simulink model "iscrt"  (R2025a)
settings: Solver=FixedStepDiscrete  StartTime=0.0  StopTime=6  FixedStep=Ts  RelTol=1e-3
model workspace (MATLAB code in the model file):
  | N = 31;
  | n = 0:N-1;
  | sigma = (N-1)/6;
  | g = exp(-0.5*((n-(N-1)/2)/sigma).^2);
  | h = g / sum(g);
undefined symbols (not defined in the file): DiscIntNeverNeededParam, Ts
libraries: simulink x2
settings Model: Creator=wattanakhonvipanna  LastModifiedBy=wattanakhonvipanna

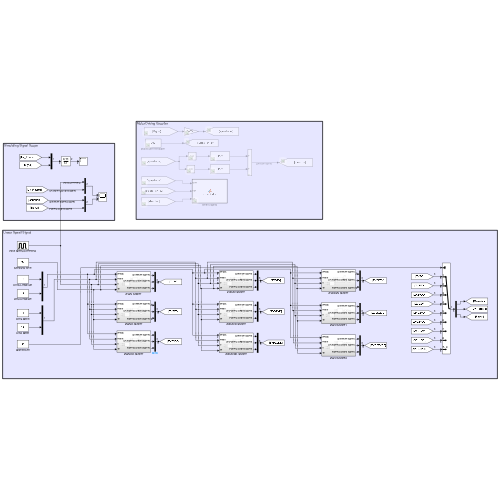
[thumbnail: Simulink's stored preview of the top-level diagram]
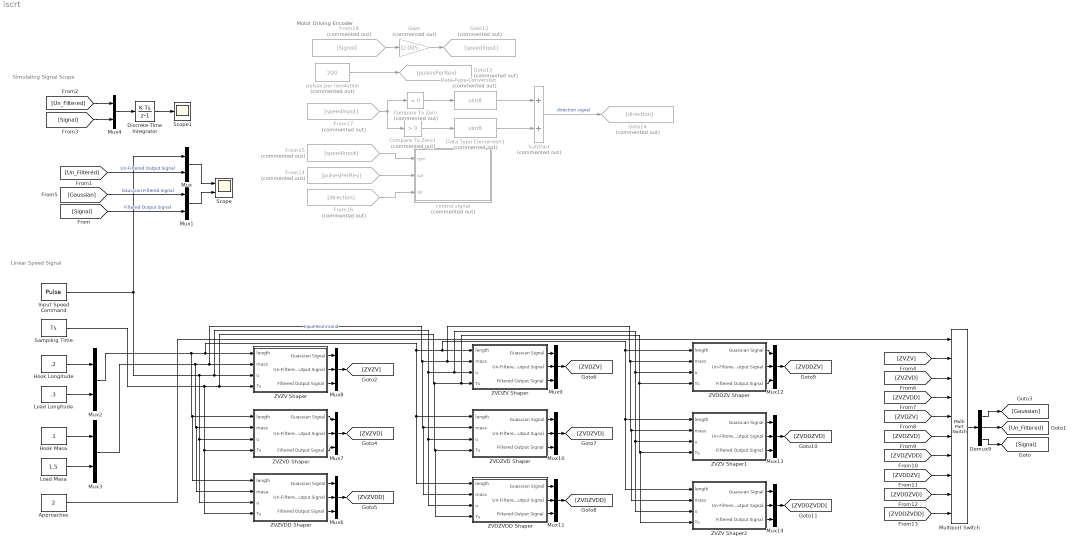
== system iscrt ==
  note: Motor Driving Encoder
  note: Linear Speed Signal
  note: Simulating Signal Scope
  Approaches : Constant  Value=2
  Compare To Zero : simulink/Logic and Bit Operations/Compare To Zero  Commented=on  relop=<  OutDataTypeStr=boolean
  Compare To Zero1 : simulink/Logic and Bit Operations/Compare To Zero  Commented=on  relop=>  OutDataTypeStr=boolean
  Data Type Conversion : DataTypeConversion  Commented=on  OutDataTypeStr=uint8  SaturateOnIntegerOverflow=off  RndMeth=Floor
  Data Type Conversion1 : DataTypeConversion  Commented=on  OutDataTypeStr=uint8  SaturateOnIntegerOverflow=off  RndMeth=Floor
  Demux9 : Demux  Outputs=3
  Discrete-Time Integrator : DiscreteIntegrator  SampleTime=-1  ICPrevOutput=DiscIntNeverNeededParam  ICPrevScaledInput=DiscIntNeverNeededParam
  From14 : From  Commented=on  GotoTag=pulsesPerRev
  From15 : From  Commented=on  GotoTag=speedInput
  From16 : From  Commented=on  GotoTag=direction
  From17 : From  Commented=on  GotoTag=speedInput
  From18 : From  Commented=on  GotoTag=Signal
  Gain : Gain  Commented=on  Gain=1/.005
  Goto12 : Goto  Commented=on  GotoTag=speedInput
  Goto13 : Goto  Commented=on  GotoTag=pulsesPerRev
  Goto14 : Goto  Commented=on  GotoTag=direction
  Hook Longitude : Constant  Value=.2
  Hook Masa : Constant  Value=.1
  Input Speed Command : DiscretePulseGenerator  PulseType=Time based  Amplitude=0.2  Period=10  PulseWidth=50
  Load Longitude : Constant  Value=.3
  Load Masa : Constant  Value=1.5
  Multiport Switch : MultiPortSwitch  Inputs=9  SaturateOnIntegerOverflow=off  InputSameDT=off
  Mux{,1..4} (5 alike) : Mux  Inputs=2
  Mux{6..14} (9 alike) : Mux  Inputs=3
  Sampling Time : Constant  Value=Ts
  Scope : Scope  NumInputPorts=2
      settings: ActiveDisplayYMinimum=-0.024999999999999994  ActiveDisplayYMaximum=0.225  YLabel=speed (m/s)
  Scope1 : Scope
      settings: ActiveDisplayYMinimum=-0.31249999999999656  ActiveDisplayYMaximum=2.8124999999999694  YLabel=position (m)  DataLoggingVariableName=ScopeData2
  Subtract : Sum  Commented=on
  ZVDDZV Shaper : Subsystem
  ZVDZV Shaper : Subsystem
  ZVDZVD Shaper : Subsystem
  ZVDZVDD Shaper : Subsystem
  ZVZV Shaper : Subsystem
  ZVZV Shaper1 : Subsystem
  ZVZV Shaper2 : Subsystem
  ZVZVD Shaper : Subsystem
  ZVZVDD Shaper : Subsystem
  control signal : MATLAB Function  Commented=on  TreatAsAtomicUnit=on
  pulses per revolution : Constant  Commented=on  Value=200
  wires:
  [Un_Filtered] -> Mux/2  "Un-Filtered Output Signal"
  Mux/1 -> Scope/1
  Input Speed Command/1 -> ZVZVDD Shaper/3(u), ZVZVD Shaper/3(u), ZVDZVDD Shaper/3(u), ZVDZVD Shaper/3(u), ZVZV Shaper2/3(u), ZVZV Shaper1/3(u), ZVDDZV Shaper/3(u), ZVDZV Shaper/3(u), ZVZV Shaper/3(u), Mux/1  "Input Command"
  [Gaussian] -> Mux1/1  "Gaussian Filtered Signal"
  [Signal] -> Mux1/2  "Filtered Output Signal"
  Hook Longitude/1 -> Mux2/1
  Load Longitude/1 -> Mux2/2
  Load Masa/1 -> Mux3/2
  Hook Masa/1 -> Mux3/1
  Mux4/1 -> Discrete-Time Integrator/1
  [Un_Filtered] -> Mux4/1
  [Signal] -> Mux4/2
  Discrete-Time Integrator/1 -> Scope1/1
  Mux3/1 -> ZVZVDD Shaper/2(masa), ZVZVD Shaper/2(mass), ZVDZVDD Shaper/2(mass), ZVDZVD Shaper/2(mass), ZVZV Shaper2/2(mass), ZVZV Shaper1/2(mass), ZVDDZV Shaper/2(mass), ZVDZV Shaper/2(mass), ZVZV Shaper/2(mass)
  Sampling Time/1 -> ZVZVDD Shaper/4(Ts), ZVZVD Shaper/4(Ts), ZVDZVDD Shaper/4(Ts), ZVDZVD Shaper/4(Ts), ZVZV Shaper2/4(Ts), ZVZV Shaper1/4(Ts), ZVDDZV Shaper/4(Ts), ZVDZV Shaper/4(Ts), ZVZV Shaper/4(Ts)
  Mux2/1 -> ZVZVDD Shaper/1(length), ZVZVD Shaper/1(length), ZVDZVDD Shaper/1(length), ZVDZVD Shaper/1(length), ZVZV Shaper2/1(length), ZVZV Shaper1/1(length), ZVDDZV Shaper/1(length), ZVDZV Shaper/1(length), ZVZV Shaper/1(length)
  ZVZVDD Shaper/2(Un-Filtered Output Signal) -> Mux6/2
  ZVZVDD Shaper/3(Filtered Output Signal) -> Mux6/3
  ZVZVDD Shaper/1(Guassian Signal) -> Mux6/1
  ZVZVD Shaper/3(Filtered Output Signal) -> Mux7/3
  ZVZVD Shaper/2(Un-Filtered Output Signal) -> Mux7/2
  ZVZVD Shaper/1(Guassian Signal) -> Mux7/1
  ZVZV Shaper/3(Filtered Output Signal) -> Mux8/3
  ZVZV Shaper/2(Un-Filtered Output Signal) -> Mux8/2
  ZVZV Shaper/1(Guassian Signal) -> Mux8/1
  ZVDZV Shaper/3(Filtered Output Signal) -> Mux9/3
  ZVDZV Shaper/2(Un-Filtered Output Signal) -> Mux9/2
  ZVDZV Shaper/1(Guassian Signal) -> Mux9/1
  ZVDZVD Shaper/1(Guassian Signal) -> Mux10/1
  ZVDZVD Shaper/2(Un-Filtered Output Signal) -> Mux10/2
  ZVDZVD Shaper/3(Filtered Output Signal) -> Mux10/3
  ZVDZVDD Shaper/1(Guassian Signal) -> Mux11/1
  ZVDZVDD Shaper/2(Un-Filtered Output Signal) -> Mux11/2
  ZVDZVDD Shaper/3(Filtered Output Signal) -> Mux11/3
  ZVDDZV Shaper/1(Guassian Signal) -> Mux12/1
  ZVDDZV Shaper/2(Un-Filtered Output Signal) -> Mux12/2
  ZVDDZV Shaper/3(Filtered Output Signal) -> Mux12/3
  ZVZV Shaper1/1(Guassian Signal) -> Mux13/1
  ZVZV Shaper1/2(Un-Filtered Output Signal) -> Mux13/2
  ZVZV Shaper1/3(Filtered Output Signal) -> Mux13/3
  ZVZV Shaper2/1(Guassian Signal) -> Mux14/1
  ZVZV Shaper2/2(Un-Filtered Output Signal) -> Mux14/2
  ZVZV Shaper2/3(Filtered Output Signal) -> Mux14/3
  Multiport Switch/1 -> Demux9/1
  Demux9/1 -> [Gaussian]
  Demux9/2 -> [Un_Filtered]
  Demux9/3 -> [Signal]
  Mux8/1 -> [ZVZV]
  Mux7/1 -> [ZVZVD]
  Mux6/1 -> [ZVZVDD]
  Mux9/1 -> [ZVDZV]
  Mux10/1 -> [ZVDZVD]
  Mux11/1 -> [ZVDZVDD]
  Mux12/1 -> [ZVDDZV]
  Mux13/1 -> [ZVDDZVD]
  Mux14/1 -> [ZVDDZVDD]
  [ZVZV] -> Multiport Switch/2
  [ZVZVD] -> Multiport Switch/3
  [ZVZVDD] -> Multiport Switch/4
  [ZVDZV] -> Multiport Switch/5
  [ZVDZVD] -> Multiport Switch/6
  [ZVDZVDD] -> Multiport Switch/7
  [ZVDDZV] -> Multiport Switch/8
  [ZVDDZVD] -> Multiport Switch/9
  [ZVDDZVDD] -> Multiport Switch/10
  Approaches/1 -> Multiport Switch/1
  Data Type Conversion/1 -> Subtract/1
  pulses per revolution/1 -> Goto13/1
  Compare To Zero/1 -> Data Type Conversion/1
  From16/1 -> control signal/3(dir)
  From15/1 -> control signal/1(rpm)
  From14/1 -> control signal/2(spr)
  Data Type Conversion1/1 -> Subtract/2
  From18/1 -> Gain/1
  Subtract/1 -> Goto14/1  "direction signal"
  Compare To Zero1/1 -> Data Type Conversion1/1
  From17/1 -> Compare To Zero/1, Compare To Zero1/1
  Gain/1 -> Goto12/1
  Mux1/1 -> Scope/2

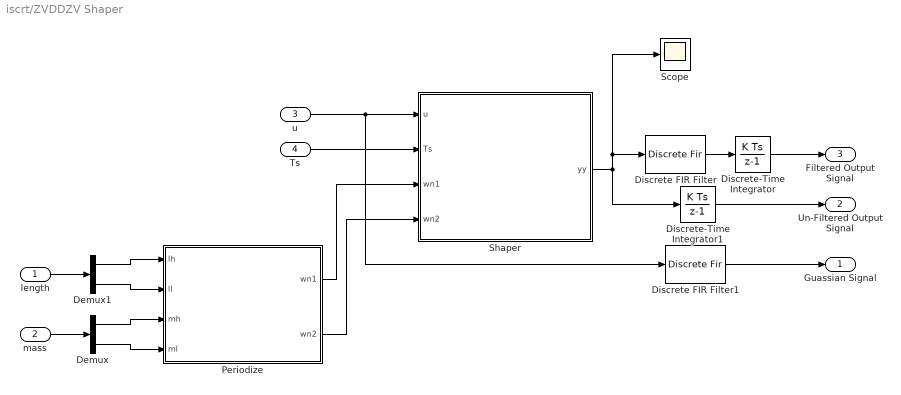
== system iscrt/ZVDDZV Shaper ==
  length : Inport
  mass : Inport  Port=2
  u : Inport  Port=3
  Ts : Inport  Port=4
  Demux : Demux  Outputs=2
  Demux1 : Demux  Outputs=2
  Discrete FIR Filter : DiscreteFir  Coefficients=h
  Discrete FIR Filter1 : DiscreteFir  Coefficients=h
  Discrete-Time Integrator : DiscreteIntegrator  SampleTime=Ts  ICPrevOutput=DiscIntNeverNeededParam  ICPrevScaledInput=DiscIntNeverNeededParam
  Discrete-Time Integrator1 : DiscreteIntegrator  SampleTime=Ts  ICPrevOutput=DiscIntNeverNeededParam  ICPrevScaledInput=DiscIntNeverNeededParam
  Periodize : MATLAB Function  TreatAsAtomicUnit=on
  Scope : Scope
      settings: ActiveDisplayYMinimum=-9993.7500000000018  ActiveDisplayYMaximum=9993.7500000000018  YLabel=Shaper Impulse (ms^-^2)
  Shaper : MATLAB Function  TreatAsAtomicUnit=on
  Guassian Signal : Outport
  Un-Filtered Output Signal : Outport  Port=2
  Filtered Output Signal : Outport  Port=3
  wires:
  Discrete-Time Integrator/1 -> Filtered Output Signal/1
  Shaper/1(yy) -> Discrete-Time Integrator1/1, Scope/1, Discrete FIR Filter/1
  Discrete FIR Filter/1 -> Discrete-Time Integrator/1
  Discrete-Time Integrator1/1 -> Un-Filtered Output Signal/1
  Discrete FIR Filter1/1 -> Guassian Signal/1
  Demux1/1 -> Periodize/1(lh)
  Demux1/2 -> Periodize/2(ll)
  Demux/1 -> Periodize/3(mh)
  Demux/2 -> Periodize/4(ml)
  Periodize/1(wn1) -> Shaper/3(wn1)
  Periodize/2(wn2) -> Shaper/4(wn2)
  mass/1 -> Demux/1
  length/1 -> Demux1/1
  Ts/1 -> Shaper/2(Ts)
  u/1 -> Discrete FIR Filter1/1, Shaper/1(u)

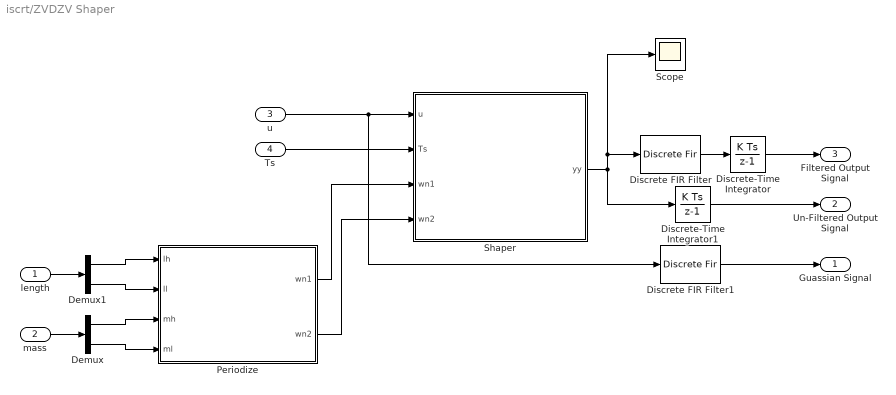
== system iscrt/ZVDZV Shaper ==
  length : Inport
  mass : Inport  Port=2
  u : Inport  Port=3
  Ts : Inport  Port=4
  Demux : Demux  Outputs=2
  Demux1 : Demux  Outputs=2
  Discrete FIR Filter : DiscreteFir  Coefficients=h
  Discrete FIR Filter1 : DiscreteFir  Coefficients=h
  Discrete-Time Integrator : DiscreteIntegrator  SampleTime=Ts  ICPrevOutput=DiscIntNeverNeededParam  ICPrevScaledInput=DiscIntNeverNeededParam
  Discrete-Time Integrator1 : DiscreteIntegrator  SampleTime=Ts  ICPrevOutput=DiscIntNeverNeededParam  ICPrevScaledInput=DiscIntNeverNeededParam
  Periodize : MATLAB Function  TreatAsAtomicUnit=on
  Scope : Scope
      settings: ActiveDisplayYMinimum=-9993.7500000000018  ActiveDisplayYMaximum=9993.7500000000018  YLabel=Shaper Impulse (ms^-^2)
  Shaper : MATLAB Function  TreatAsAtomicUnit=on
  Guassian Signal : Outport
  Un-Filtered Output Signal : Outport  Port=2
  Filtered Output Signal : Outport  Port=3
  wires:
  Discrete-Time Integrator/1 -> Filtered Output Signal/1
  Shaper/1(yy) -> Discrete-Time Integrator1/1, Scope/1, Discrete FIR Filter/1
  Discrete FIR Filter/1 -> Discrete-Time Integrator/1
  Discrete-Time Integrator1/1 -> Un-Filtered Output Signal/1
  Discrete FIR Filter1/1 -> Guassian Signal/1
  Demux1/1 -> Periodize/1(lh)
  Demux1/2 -> Periodize/2(ll)
  Demux/1 -> Periodize/3(mh)
  Demux/2 -> Periodize/4(ml)
  Periodize/1(wn1) -> Shaper/3(wn1)
  Periodize/2(wn2) -> Shaper/4(wn2)
  mass/1 -> Demux/1
  length/1 -> Demux1/1
  Ts/1 -> Shaper/2(Ts)
  u/1 -> Discrete FIR Filter1/1, Shaper/1(u)

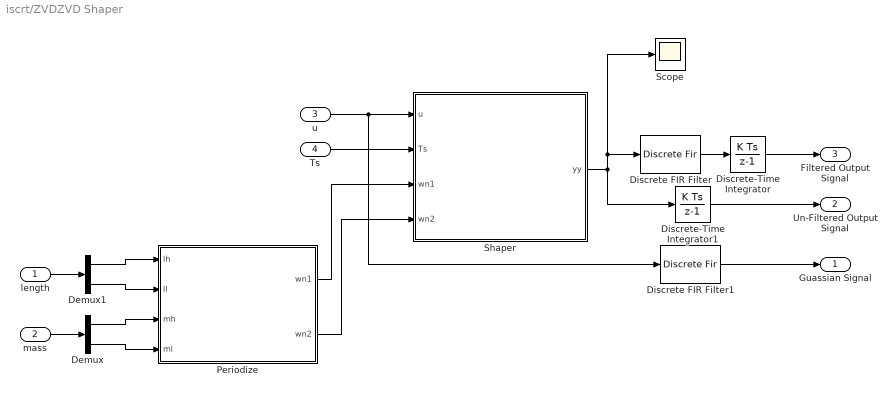
== system iscrt/ZVDZVD Shaper ==
  length : Inport
  mass : Inport  Port=2
  u : Inport  Port=3
  Ts : Inport  Port=4
  Demux : Demux  Outputs=2
  Demux1 : Demux  Outputs=2
  Discrete FIR Filter : DiscreteFir  Coefficients=h
  Discrete FIR Filter1 : DiscreteFir  Coefficients=h
  Discrete-Time Integrator : DiscreteIntegrator  SampleTime=Ts  ICPrevOutput=DiscIntNeverNeededParam  ICPrevScaledInput=DiscIntNeverNeededParam
  Discrete-Time Integrator1 : DiscreteIntegrator  SampleTime=Ts  ICPrevOutput=DiscIntNeverNeededParam  ICPrevScaledInput=DiscIntNeverNeededParam
  Periodize : MATLAB Function  TreatAsAtomicUnit=on
  Scope : Scope
      settings: ActiveDisplayYMinimum=-9993.7500000000018  ActiveDisplayYMaximum=9993.7500000000018  YLabel=Shaper Impulse (ms^-^2)
  Shaper : MATLAB Function  TreatAsAtomicUnit=on
  Guassian Signal : Outport
  Un-Filtered Output Signal : Outport  Port=2
  Filtered Output Signal : Outport  Port=3
  wires:
  Discrete-Time Integrator/1 -> Filtered Output Signal/1
  Shaper/1(yy) -> Discrete-Time Integrator1/1, Scope/1, Discrete FIR Filter/1
  Discrete FIR Filter/1 -> Discrete-Time Integrator/1
  Discrete-Time Integrator1/1 -> Un-Filtered Output Signal/1
  Discrete FIR Filter1/1 -> Guassian Signal/1
  Demux1/1 -> Periodize/1(lh)
  Demux1/2 -> Periodize/2(ll)
  Demux/1 -> Periodize/3(mh)
  Demux/2 -> Periodize/4(ml)
  Periodize/1(wn1) -> Shaper/3(wn1)
  Periodize/2(wn2) -> Shaper/4(wn2)
  length/1 -> Demux1/1
  mass/1 -> Demux/1
  Ts/1 -> Shaper/2(Ts)
  u/1 -> Discrete FIR Filter1/1, Shaper/1(u)

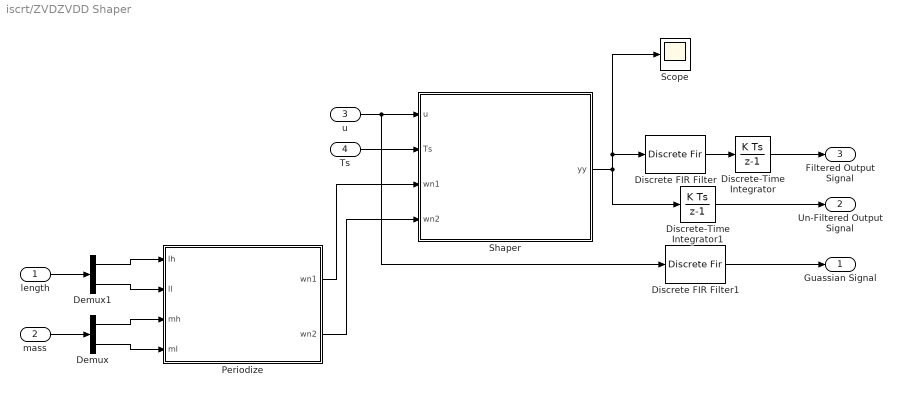
== system iscrt/ZVDZVDD Shaper ==
  length : Inport
  mass : Inport  Port=2
  u : Inport  Port=3
  Ts : Inport  Port=4
  Demux : Demux  Outputs=2
  Demux1 : Demux  Outputs=2
  Discrete FIR Filter : DiscreteFir  Coefficients=h
  Discrete FIR Filter1 : DiscreteFir  Coefficients=h
  Discrete-Time Integrator : DiscreteIntegrator  SampleTime=Ts  ICPrevOutput=DiscIntNeverNeededParam  ICPrevScaledInput=DiscIntNeverNeededParam
  Discrete-Time Integrator1 : DiscreteIntegrator  SampleTime=Ts  ICPrevOutput=DiscIntNeverNeededParam  ICPrevScaledInput=DiscIntNeverNeededParam
  Periodize : MATLAB Function  TreatAsAtomicUnit=on
  Scope : Scope
      settings: ActiveDisplayYMinimum=-9993.7500000000018  ActiveDisplayYMaximum=9993.7500000000018  YLabel=Shaper Impulse (ms^-^2)
  Shaper : MATLAB Function  TreatAsAtomicUnit=on
  Guassian Signal : Outport
  Un-Filtered Output Signal : Outport  Port=2
  Filtered Output Signal : Outport  Port=3
  wires:
  Discrete-Time Integrator/1 -> Filtered Output Signal/1
  Shaper/1(yy) -> Discrete-Time Integrator1/1, Scope/1, Discrete FIR Filter/1
  Discrete FIR Filter/1 -> Discrete-Time Integrator/1
  Discrete-Time Integrator1/1 -> Un-Filtered Output Signal/1
  Discrete FIR Filter1/1 -> Guassian Signal/1
  Demux1/1 -> Periodize/1(lh)
  Demux1/2 -> Periodize/2(ll)
  Demux/1 -> Periodize/3(mh)
  Demux/2 -> Periodize/4(ml)
  Periodize/1(wn1) -> Shaper/3(wn1)
  Periodize/2(wn2) -> Shaper/4(wn2)
  u/1 -> Discrete FIR Filter1/1, Shaper/1(u)
  Ts/1 -> Shaper/2(Ts)
  length/1 -> Demux1/1
  mass/1 -> Demux/1

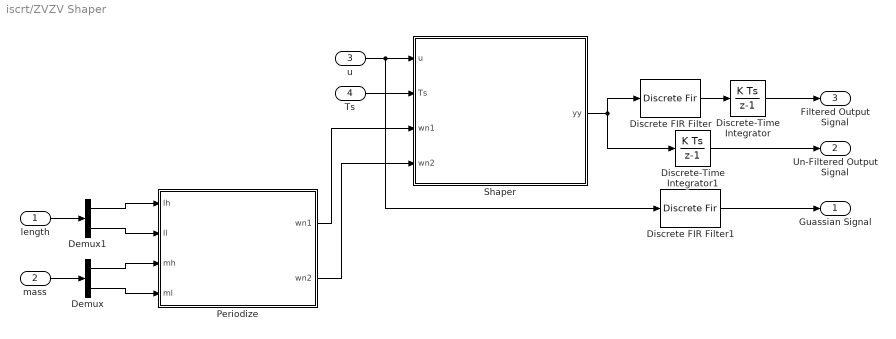
== system iscrt/ZVZV Shaper ==
  length : Inport
  mass : Inport  Port=2
  u : Inport  Port=3
  Ts : Inport  Port=4
  Demux : Demux  Outputs=2
  Demux1 : Demux  Outputs=2
  Discrete FIR Filter : DiscreteFir  Coefficients=h
  Discrete FIR Filter1 : DiscreteFir  Coefficients=h
  Discrete-Time Integrator : DiscreteIntegrator  SampleTime=Ts  ICPrevOutput=DiscIntNeverNeededParam  ICPrevScaledInput=DiscIntNeverNeededParam
  Discrete-Time Integrator1 : DiscreteIntegrator  SampleTime=Ts  ICPrevOutput=DiscIntNeverNeededParam  ICPrevScaledInput=DiscIntNeverNeededParam
  Periodize : MATLAB Function  TreatAsAtomicUnit=on
  Shaper : MATLAB Function  TreatAsAtomicUnit=on
  Guassian Signal : Outport
  Un-Filtered Output Signal : Outport  Port=2
  Filtered Output Signal : Outport  Port=3
  wires:
  Discrete-Time Integrator/1 -> Filtered Output Signal/1
  Shaper/1(yy) -> Discrete-Time Integrator1/1, Discrete FIR Filter/1
  Discrete FIR Filter/1 -> Discrete-Time Integrator/1
  Discrete-Time Integrator1/1 -> Un-Filtered Output Signal/1
  Discrete FIR Filter1/1 -> Guassian Signal/1
  Demux1/1 -> Periodize/1(lh)
  Demux1/2 -> Periodize/2(ll)
  Demux/1 -> Periodize/3(mh)
  Demux/2 -> Periodize/4(ml)
  Periodize/1(wn1) -> Shaper/3(wn1)
  Periodize/2(wn2) -> Shaper/4(wn2)
  length/1 -> Demux1/1
  mass/1 -> Demux/1
  u/1 -> Discrete FIR Filter1/1, Shaper/1(u)
  Ts/1 -> Shaper/2(Ts)

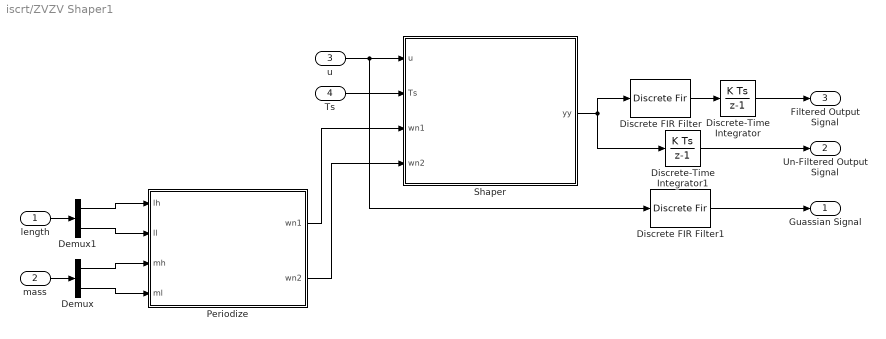
== system iscrt/ZVZV Shaper1 ==
  length : Inport
  mass : Inport  Port=2
  u : Inport  Port=3
  Ts : Inport  Port=4
  Demux : Demux  Outputs=2
  Demux1 : Demux  Outputs=2
  Discrete FIR Filter : DiscreteFir  Coefficients=h
  Discrete FIR Filter1 : DiscreteFir  Coefficients=h
  Discrete-Time Integrator : DiscreteIntegrator  SampleTime=Ts  ICPrevOutput=DiscIntNeverNeededParam  ICPrevScaledInput=DiscIntNeverNeededParam
  Discrete-Time Integrator1 : DiscreteIntegrator  SampleTime=Ts  ICPrevOutput=DiscIntNeverNeededParam  ICPrevScaledInput=DiscIntNeverNeededParam
  Periodize : MATLAB Function  TreatAsAtomicUnit=on
  Shaper : MATLAB Function  TreatAsAtomicUnit=on
  Guassian Signal : Outport
  Un-Filtered Output Signal : Outport  Port=2
  Filtered Output Signal : Outport  Port=3
  wires:
  Discrete-Time Integrator/1 -> Filtered Output Signal/1
  Shaper/1(yy) -> Discrete-Time Integrator1/1, Discrete FIR Filter/1
  Discrete FIR Filter/1 -> Discrete-Time Integrator/1
  Discrete-Time Integrator1/1 -> Un-Filtered Output Signal/1
  Discrete FIR Filter1/1 -> Guassian Signal/1
  Demux1/1 -> Periodize/1(lh)
  Demux1/2 -> Periodize/2(ll)
  Demux/1 -> Periodize/3(mh)
  Demux/2 -> Periodize/4(ml)
  Periodize/1(wn1) -> Shaper/3(wn1)
  Periodize/2(wn2) -> Shaper/4(wn2)
  u/1 -> Discrete FIR Filter1/1, Shaper/1(u)
  Ts/1 -> Shaper/2(Ts)
  mass/1 -> Demux/1
  length/1 -> Demux1/1

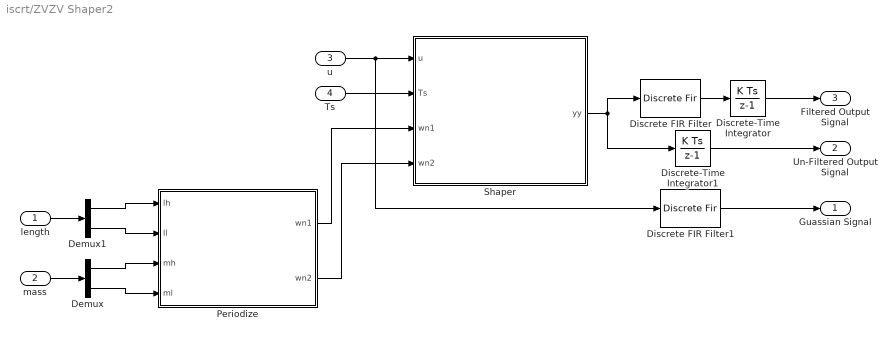
== system iscrt/ZVZV Shaper2 ==
  length : Inport
  mass : Inport  Port=2
  u : Inport  Port=3
  Ts : Inport  Port=4
  Demux : Demux  Outputs=2
  Demux1 : Demux  Outputs=2
  Discrete FIR Filter : DiscreteFir  Coefficients=h
  Discrete FIR Filter1 : DiscreteFir  Coefficients=h
  Discrete-Time Integrator : DiscreteIntegrator  SampleTime=Ts  ICPrevOutput=DiscIntNeverNeededParam  ICPrevScaledInput=DiscIntNeverNeededParam
  Discrete-Time Integrator1 : DiscreteIntegrator  SampleTime=Ts  ICPrevOutput=DiscIntNeverNeededParam  ICPrevScaledInput=DiscIntNeverNeededParam
  Periodize : MATLAB Function  TreatAsAtomicUnit=on
  Shaper : MATLAB Function  TreatAsAtomicUnit=on
  Guassian Signal : Outport
  Un-Filtered Output Signal : Outport  Port=2
  Filtered Output Signal : Outport  Port=3
  wires:
  Discrete-Time Integrator/1 -> Filtered Output Signal/1
  Shaper/1(yy) -> Discrete-Time Integrator1/1, Discrete FIR Filter/1
  Discrete FIR Filter/1 -> Discrete-Time Integrator/1
  Discrete-Time Integrator1/1 -> Un-Filtered Output Signal/1
  Discrete FIR Filter1/1 -> Guassian Signal/1
  Demux1/1 -> Periodize/1(lh)
  Demux1/2 -> Periodize/2(ll)
  Demux/1 -> Periodize/3(mh)
  Demux/2 -> Periodize/4(ml)
  Periodize/1(wn1) -> Shaper/3(wn1)
  Periodize/2(wn2) -> Shaper/4(wn2)
  Ts/1 -> Shaper/2(Ts)
  length/1 -> Demux1/1
  mass/1 -> Demux/1
  u/1 -> Discrete FIR Filter1/1, Shaper/1(u)

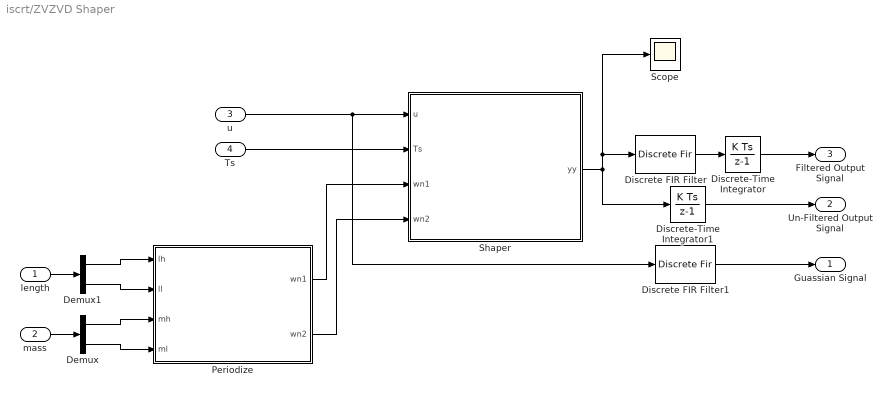
== system iscrt/ZVZVD Shaper ==
  length : Inport
  mass : Inport  Port=2
  u : Inport  Port=3
  Ts : Inport  Port=4
  Demux : Demux  Outputs=2
  Demux1 : Demux  Outputs=2
  Discrete FIR Filter : DiscreteFir  Coefficients=h
  Discrete FIR Filter1 : DiscreteFir  Coefficients=h
  Discrete-Time Integrator : DiscreteIntegrator  SampleTime=Ts  ICPrevOutput=DiscIntNeverNeededParam  ICPrevScaledInput=DiscIntNeverNeededParam
  Discrete-Time Integrator1 : DiscreteIntegrator  SampleTime=Ts  ICPrevOutput=DiscIntNeverNeededParam  ICPrevScaledInput=DiscIntNeverNeededParam
  Periodize : MATLAB Function  TreatAsAtomicUnit=on
  Scope : Scope
      settings: ActiveDisplayYMinimum=-1332.5  ActiveDisplayYMaximum=1332.5  YLabel=Shaper Impulse (ms^-^2)
  Shaper : MATLAB Function  TreatAsAtomicUnit=on
  Guassian Signal : Outport
  Un-Filtered Output Signal : Outport  Port=2
  Filtered Output Signal : Outport  Port=3
  wires:
  Discrete-Time Integrator/1 -> Filtered Output Signal/1
  Shaper/1(yy) -> Discrete-Time Integrator1/1, Scope/1, Discrete FIR Filter/1
  Discrete FIR Filter/1 -> Discrete-Time Integrator/1
  Discrete-Time Integrator1/1 -> Un-Filtered Output Signal/1
  Discrete FIR Filter1/1 -> Guassian Signal/1
  Demux1/1 -> Periodize/1(lh)
  Demux1/2 -> Periodize/2(ll)
  Demux/1 -> Periodize/3(mh)
  Demux/2 -> Periodize/4(ml)
  Periodize/1(wn1) -> Shaper/3(wn1)
  Periodize/2(wn2) -> Shaper/4(wn2)
  mass/1 -> Demux/1
  length/1 -> Demux1/1
  Ts/1 -> Shaper/2(Ts)
  u/1 -> Discrete FIR Filter1/1, Shaper/1(u)

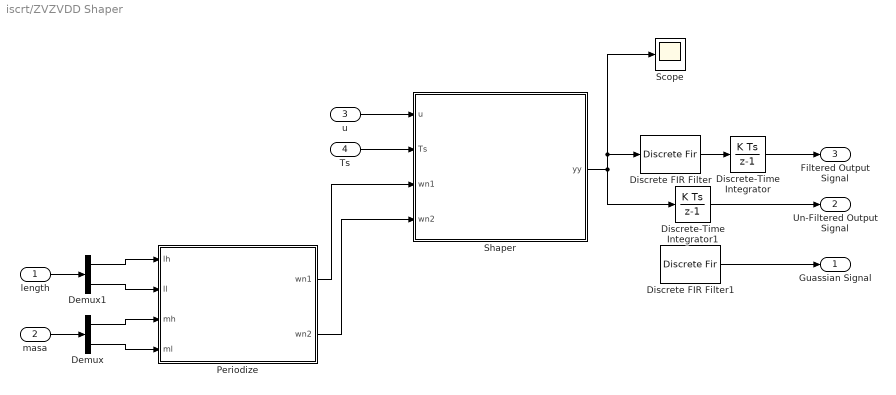
== system iscrt/ZVZVDD Shaper ==
  length : Inport
  masa : Inport  Port=2
  u : Inport  Port=3
  Ts : Inport  Port=4
  Demux : Demux  Outputs=2
  Demux1 : Demux  Outputs=2
  Discrete FIR Filter : DiscreteFir  Coefficients=h
  Discrete FIR Filter1 : DiscreteFir  Coefficients=h
  Discrete-Time Integrator : DiscreteIntegrator  SampleTime=Ts  ICPrevOutput=DiscIntNeverNeededParam  ICPrevScaledInput=DiscIntNeverNeededParam
  Discrete-Time Integrator1 : DiscreteIntegrator  SampleTime=Ts  ICPrevOutput=DiscIntNeverNeededParam  ICPrevScaledInput=DiscIntNeverNeededParam
  Periodize : MATLAB Function  TreatAsAtomicUnit=on
  Scope : Scope
      settings: ActiveDisplayYMinimum=-9993.7500000000018  ActiveDisplayYMaximum=9993.7500000000018  YLabel=Shaper Impulse (ms^-^2)
  Shaper : MATLAB Function  TreatAsAtomicUnit=on
  Guassian Signal : Outport
  Un-Filtered Output Signal : Outport  Port=2
  Filtered Output Signal : Outport  Port=3
  wires:
  Discrete-Time Integrator/1 -> Filtered Output Signal/1
  Shaper/1(yy) -> Discrete-Time Integrator1/1, Scope/1, Discrete FIR Filter/1
  Discrete FIR Filter/1 -> Discrete-Time Integrator/1
  Discrete-Time Integrator1/1 -> Un-Filtered Output Signal/1
  Discrete FIR Filter1/1 -> Guassian Signal/1
  Demux1/1 -> Periodize/1(lh)
  Demux1/2 -> Periodize/2(ll)
  Demux/1 -> Periodize/3(mh)
  Demux/2 -> Periodize/4(ml)
  Periodize/1(wn1) -> Shaper/3(wn1)
  Periodize/2(wn2) -> Shaper/4(wn2)
  masa/1 -> Demux/1
  length/1 -> Demux1/1
  u/1 -> Shaper/1(u)
  Ts/1 -> Shaper/2(Ts)

== matlab function iscrt/ZVDZVD Shaper/Shaper ==
  data: u input; yy output; Ts input; wn1 input; wn2 input
function yy = ZVZVshaper(u, Ts, wn1, wn2)

persistent armed k last_u A_tot d2 d3 d4 d5 d6 d7 d8 d9
if isempty(armed)
    armed  = false;
    k      = double(0);
    last_u = 0.0;
    A_tot  = 0.0;
    d2     = double(0);
    d3     = double(0);
    d4     = double(0);
    d5     = double(0);
    d6     = double(0);
    d7     = double(0);
    d8     = double(0);
    d9     = double(0);
end

yy = 0.0;                
tol = 1e-12;

du = u - last_u;
last_u = u;

if ~armed && (abs(du) > tol)
    A_tot = du;
    k     = double(0);
    T1    = 2*pi / max(wn1, 1e-9);
    T2    = 2*pi / max(wn2, 1e-9);
    d2    = double( round( (0.5*T2) / max(Ts,1e-12) ) ); 
    d3    = double( round( T2 / max(Ts,1e-12) ) );
    d4    = double( round( (0.5*T1) / max(Ts,1e-12) ) );
    d5    = double( round( 0.5*(T1+T2) / max(Ts,1e-12) ) );
    d6    = double( round( (0.5*T1+T2) / max(Ts,1e-12) ) );
    d7    = double( round( T1 / max(Ts,1e-12) ) );
    d8    = double( round( (0.5*T2+T1) / max(Ts,1e-12) ) );
    d9    = double( round( (T2+T1) / max(Ts,1e-12) ) );
    armed = true;
end


if armed
    if k == double(0)
        yy = ((1/16)*A_tot)  / max(Ts,1e-12);
    elseif k == d2
        yy = ((2/16)*A_tot)  / max(Ts,1e-12);
    elseif k == d3
        yy = ((1/16)*A_tot)  / max(Ts,1e-12);
    elseif k == d4
        yy = ((2/16)*A_tot)  / max(Ts,1e-12);
    elseif k == d5
        yy = ((4/16)*A_tot)  / max(Ts,1e-12);
    elseif k == d6
        yy = ((2/16)*A_tot)  / max(Ts,1e-12);
    elseif k == d7
        yy = ((1/16)*A_tot)  / max(Ts,1e-12);
    elseif k == d8
        yy = ((2/16)*A_tot)  / max(Ts,1e-12);
    elseif k == d9
        yy = ((1/16)*A_tot)  / max(Ts,1e-12);
    end

    k = k + double(1);
    if k > d9 + double(1)
        armed = false;
    end
end

== matlab function iscrt/ZVDZVDD Shaper/Periodize ==
  data: lh input; ll input; mh input; wn1 output; wn2 output; ml input
function [wn1, wn2]= ModePeriodize(lh, ll, mh, ml)

g = 9.81;

a = mh * lh * ll;
b = (mh * g * ll) + (ml * g * ll) + (mh * g * lh) + (ml * g * lh);
c = (mh * g * g) + (ml * g * g);

wn1 = sqrt((b - sqrt(b * b - 4 * a * c))/ (2 * a));
wn2 = sqrt((b + sqrt(b * b - 4 * a * c))/ (2 * a));

== matlab function iscrt/ZVDZVDD Shaper/Shaper ==
  data: u input; yy output; Ts input; wn1 input; wn2 input
function yy = ZVZVshaper(u, Ts, wn1, wn2)

persistent armed k last_u A_tot d2 d3 d4 d5 d6 d7 d8 d9 d10 d11 d12
if isempty(armed)
    armed  = false;
    k      = double(0);
    last_u = 0.0;
    A_tot  = 0.0;
    d2     = double(0);
    d3     = double(0);
    d4     = double(0);
    d5     = double(0);
    d6     = double(0);
    d7     = double(0);
    d8     = double(0);
    d9     = double(0);
    d10    = double(0);
    d11    = double(0);
    d12    = double(0);
end

yy = 0.0;                
tol = 1e-12;

du = u - last_u;
last_u = u;

if ~armed && (abs(du) > tol)
    A_tot = du;
    k     = double(0);
    T1    = 2*pi / max(wn1, 1e-9);
    T2    = 2*pi / max(wn2, 1e-9);
    d2    = double( round( (0.5*T2) / max(Ts,1e-12) ) ); 
    d3    = double( round( T2 / max(Ts,1e-12) ) );
    d4    = double( round( (1.5*T2) / max(Ts,1e-12) ) );
    d5    = double( round( (0.5*T1) / max(Ts,1e-12) ) );
    d6    = double( round( 0.5*(T1+T2) / max(Ts,1e-12) ) );
    d7    = double( round( (0.5*T1+T2) / max(Ts,1e-12) ) );
    d8    = double( round( (0.5*T1+1.5*T2) / max(Ts,1e-12) ) );
    d9    = double( round( T1 / max(Ts,1e-12) ) );
    d10   = double( round( (0.5*T2+T1) / max(Ts,1e-12) ) );
    d11   = double( round( (T1+T2) / max(Ts,1e-12) ) );
    d12   = double( round( (T1+1.5*T2) / max(Ts,1e-12) ) );
    armed = true;
end


if armed
    if k == double(0)
        yy = ((1/32)*A_tot)  / max(Ts,1e-12);
    elseif k == d2
        yy = ((3/32)*A_tot)  / max(Ts,1e-12);
    elseif k == d3
        yy = ((3/32)*A_tot)  / max(Ts,1e-12);
    elseif k == d4
        yy = ((1/32)*A_tot)  / max(Ts,1e-12);
    elseif k == d5
        yy = ((2/32)*A_tot)  / max(Ts,1e-12);
    elseif k == d6
        yy = ((6/32)*A_tot)  / max(Ts,1e-12);
    elseif k == d7
        yy = ((6/32)*A_tot)  / max(Ts,1e-12);
    elseif k == d8
        yy = ((2/32)*A_tot)  / max(Ts,1e-12);
    elseif k == d9
        yy = ((1/32)*A_tot)  / max(Ts,1e-12);
    elseif k == d10
        yy = ((3/32)*A_tot)  / max(Ts,1e-12);
    elseif k == d11
        yy = ((3/32)*A_tot)  / max(Ts,1e-12);
    elseif k == d12
        yy = ((1/32)*A_tot)  / max(Ts,1e-12);
    end

    k = k + double(1);
    if k > d12 + double(1)
        armed = false;
    end
end

== matlab function iscrt/ZVZV Shaper/Periodize ==
  data: lh input; ll input; mh input; wn1 output; wn2 output; ml input
function [wn1, wn2]= ModePeriodize(lh, ll, mh, ml)

g = 9.81;

a = mh * lh * ll;
b = (mh * g * ll) + (ml * g * ll) + (mh * g * lh) + (ml * g * lh);
c = (mh * g * g) + (ml * g * g);

wn1 = sqrt((b - sqrt(b * b - 4 * a * c))/ (2 * a));
wn2 = sqrt((b + sqrt(b * b - 4 * a * c))/ (2 * a));

== matlab function iscrt/ZVDDZV Shaper/Periodize ==
  data: lh input; ll input; mh input; wn1 output; wn2 output; ml input
function [wn1, wn2]= ModePeriodize(lh, ll, mh, ml)

g = 9.81;

a = mh * lh * ll;
b = (mh * g * ll) + (ml * g * ll) + (mh * g * lh) + (ml * g * lh);
c = (mh * g * g) + (ml * g * g);

wn1 = sqrt((b - sqrt(b * b - 4 * a * c))/ (2 * a));
wn2 = sqrt((b + sqrt(b * b - 4 * a * c))/ (2 * a));

== matlab function iscrt/ZVDDZV Shaper/Shaper ==
  data: u input; yy output; Ts input; wn1 input; wn2 input
function yy = ZVZVshaper(u, Ts, wn1, wn2)

persistent armed k last_u A_tot d2 d3 d4 d5 d6 d7 d8
if isempty(armed)
    armed  = false;
    k      = double(0);
    last_u = 0.0;
    A_tot  = 0.0;
    d2     = double(0);
    d3     = double(0);
    d4     = double(0);
    d5     = double(0);
    d6     = double(0);
    d7     = double(0);
    d8     = double(0);
end

yy = 0.0;                
tol = 1e-12;

du = u - last_u;
last_u = u;

if ~armed && (abs(du) > tol)
    A_tot = du;
    k     = double(0);
    T1    = 2*pi / max(wn1, 1e-9);
    T2    = 2*pi / max(wn2, 1e-9);
    d2    = double( round( (0.5*T2) / max(Ts,1e-12) ) ); 
    d3    = double( round( (0.5*T1) / max(Ts,1e-12) ) );
    d4    = double( round( 0.5*(T1+T2) / max(Ts,1e-12) ) );
    d5    = double( round( T1 / max(Ts,1e-12) ) );
    d6    = double( round( (0.5*T2+T1) / max(Ts,1e-12) ) );
    d7    = double( round( (1.5*T1) / max(Ts,1e-12) ) );
    d8    = double( round( ((1.5*T1)+(0.5*T2)) / max(Ts,1e-12) ) );
    armed = true;
end


if armed
    if k == double(0)
        yy = ((1/16)*A_tot)  / max(Ts,1e-12);
    elseif k == d2
        yy = ((1/16)*A_tot)  / max(Ts,1e-12);
    elseif k == d3
        yy = ((3/16)*A_tot)  / max(Ts,1e-12);
    elseif k == d4
        yy = ((3/16)*A_tot)  / max(Ts,1e-12);
    elseif k == d5
        yy = ((3/16)*A_tot)  / max(Ts,1e-12);
    elseif k == d6
        yy = ((3/16)*A_tot)  / max(Ts,1e-12);
    elseif k == d7
        yy = ((1/16)*A_tot)  / max(Ts,1e-12);
    elseif k == d8
        yy = ((1/16)*A_tot)  / max(Ts,1e-12);
    end

    k = k + double(1);
    if k > d8 + double(1)
        armed = false;
    end
end

== matlab function iscrt/ZVZV Shaper1/Periodize ==
  data: lh input; ll input; mh input; wn1 output; wn2 output; ml input
function [wn1, wn2]= ModePeriodize(lh, ll, mh, ml)

g = 9.81;

a = mh * lh * ll;
b = (mh * g * ll) + (ml * g * ll) + (mh * g * lh) + (ml * g * lh);
c = (mh * g * g) + (ml * g * g);

wn1 = sqrt((b - sqrt(b * b - 4 * a * c))/ (2 * a));
wn2 = sqrt((b + sqrt(b * b - 4 * a * c))/ (2 * a));

== matlab function iscrt/ZVZV Shaper1/Shaper ==
  data: u input; yy output; Ts input; wn1 input; wn2 input
function yy = ZVZVshaper(u, Ts, wn1, wn2)

persistent armed k last_u A_tot d2 d3 d4 d5 d6 d7 d8 d9 d10 d11 d12
if isempty(armed)
    armed  = false;
    k      = double(0);
    last_u = 0.0;
    A_tot  = 0.0;
    d2     = double(0);
    d3     = double(0);
    d4     = double(0);
    d5     = double(0);
    d6     = double(0);
    d7     = double(0);
    d8     = double(0);
    d9     = double(0);
    d10    = double(0);
    d11    = double(0);
    d12    = double(0);
end

yy = 0.0;                
tol = 1e-12;

du = u - last_u;
last_u = u;

if ~armed && (abs(du) > tol)
    A_tot = du;
    k     = double(0);
    T1    = 2*pi / max(wn1, 1e-9);
    T2    = 2*pi / max(wn2, 1e-9);
    d2    = double( round( (0.5*T2) / max(Ts,1e-12) ) ); 
    d3    = double( round( T2 / max(Ts,1e-12) ) );
    d4    = double( round( (0.5*T1) / max(Ts,1e-12) ) );
    d5    = double( round( 0.5*(T1+T2) / max(Ts,1e-12) ) );
    d6    = double( round( (0.5*T1+T2) / max(Ts,1e-12) ) );
    d7    = double( round( T1 / max(Ts,1e-12) ) );
    d8    = double( round( (T1+0.5*T2) / max(Ts,1e-12) ) );
    d9    = double( round( (T1+T2) / max(Ts,1e-12) ) );
    d10   = double( round( (1.5*T1) / max(Ts,1e-12) ) );
    d11   = double( round( (1.5*T1+0.5*T2) / max(Ts,1e-12) ) );
    d12   = double( round( (1.5*T1+T2) / max(Ts,1e-12) ) );
    armed = true;
end


if armed
    if k == double(0)
        yy = ((1/32)*A_tot)  / max(Ts,1e-12);
    elseif k == d2
        yy = ((2/32)*A_tot)  / max(Ts,1e-12);
    elseif k == d3
        yy = ((1/32)*A_tot)  / max(Ts,1e-12);
    elseif k == d4
        yy = ((3/32)*A_tot)  / max(Ts,1e-12);
    elseif k == d5
        yy = ((6/32)*A_tot)  / max(Ts,1e-12);
    elseif k == d6
        yy = ((3/32)*A_tot)  / max(Ts,1e-12);
    elseif k == d7
        yy = ((3/32)*A_tot)  / max(Ts,1e-12);
    elseif k == d8
        yy = ((6/32)*A_tot)  / max(Ts,1e-12);
    elseif k == d9
        yy = ((3/32)*A_tot)  / max(Ts,1e-12);
    elseif k == d10
        yy = ((1/32)*A_tot)  / max(Ts,1e-12);
    elseif k == d11
        yy = ((2/32)*A_tot)  / max(Ts,1e-12);
    elseif k == d12
        yy = ((1/32)*A_tot)  / max(Ts,1e-12);
    end

    k = k + double(1);
    if k > d12 + double(1)
        armed = false;
    end
end

== matlab function iscrt/ZVZV Shaper2/Periodize ==
  data: lh input; ll input; mh input; wn1 output; wn2 output; ml input
function [wn1, wn2]= ModePeriodize(lh, ll, mh, ml)

g = 9.81;

a = mh * lh * ll;
b = (mh * g * ll) + (ml * g * ll) + (mh * g * lh) + (ml * g * lh);
c = (mh * g * g) + (ml * g * g);

wn1 = sqrt((b - sqrt(b * b - 4 * a * c))/ (2 * a));
wn2 = sqrt((b + sqrt(b * b - 4 * a * c))/ (2 * a));

== matlab function iscrt/ZVZV Shaper2/Shaper ==
  data: u input; yy output; Ts input; wn1 input; wn2 input
function yy = ZVZVshaper(u, Ts, wn1, wn2)

persistent armed k last_u A_tot d2 d3 d4 d5 d6 d7 d8 d9 d10 d11 d12 d13 ...
    d14 d15 d16
if isempty(armed)
    armed  = false;
    k      = double(0);
    last_u = 0.0;
    A_tot  = 0.0;
    d2     = double(0);
    d3     = double(0);
    d4     = double(0);
    d5     = double(0);
    d6     = double(0);
    d7     = double(0);
    d8     = double(0);
    d9     = double(0);
    d10    = double(0);
    d11    = double(0);
    d12    = double(0);
    d13    = double(0);
    d14    = double(0);
    d15    = double(0);
    d16    = double(0);

end

yy = 0.0;                
tol = 1e-12;

du = u - last_u;
last_u = u;

if ~armed && (abs(du) > tol)
    A_tot = du;
    k     = double(0);
    T1    = 2*pi / max(wn1, 1e-9);
    T2    = 2*pi / max(wn2, 1e-9);
    d2    = double( round( (0.5*T2) / max(Ts,1e-12) ) ); 
    d3    = double( round( T2 / max(Ts,1e-12) ) );
    d4    = double( round( (1.5*T2) / max(Ts,1e-12) ) );
    d5    = double( round( (0.5*T1) / max(Ts,1e-12) ) );
    d6    = double( round( 0.5*(T1+T2) / max(Ts,1e-12) ) );
    d7    = double( round( (0.5*T1+T2) / max(Ts,1e-12) ) );
    d8    = double( round( T1 / max(Ts,1e-12) ) );
    d9    = double( round( (T1+0.5*T2) / max(Ts,1e-12) ) );
    d10   = double( round( (T1+T2) / max(Ts,1e-12) ) );
    d11   = double( round( (T1+1.5*T2) / max(Ts,1e-12) ) );
    d12   = double( round( (1.5*T1) / max(Ts,1e-12) ) );
    d13   = double( round( (1.5*T1+0.5*T2) / max(Ts,1e-12) ) );
    d14   = double( round( (1.5*T1+T2) / max(Ts,1e-12) ) );
    d15   = double( round( (1.5*T1+T2) / max(Ts,1e-12) ) );
    d16   = double( round( (1.5*T1+1.5*T2) / max(Ts,1e-12) ) );
    armed = true;
end


if armed
    if k == double(0)
        yy = ((1/64)*A_tot)  / max(Ts,1e-12);
    elseif k == d2
        yy = ((3/64)*A_tot)  / max(Ts,1e-12);
    elseif k == d3
        yy = ((3/64)*A_tot)  / max(Ts,1e-12);
    elseif k == d4
        yy = ((1/64)*A_tot)  / max(Ts,1e-12);
    elseif k == d5
        yy = ((3/64)*A_tot)  / max(Ts,1e-12);
    elseif k == d6
        yy = ((9/64)*A_tot)  / max(Ts,1e-12);
    elseif k == d7
        yy = ((9/64)*A_tot)  / max(Ts,1e-12);
    elseif k == d8
        yy = ((3/64)*A_tot)  / max(Ts,1e-12);
    elseif k == d9
        yy = ((3/64)*A_tot)  / max(Ts,1e-12);
    elseif k == d10
        yy = ((9/64)*A_tot)  / max(Ts,1e-12);
    elseif k == d11
        yy = ((9/64)*A_tot)  / max(Ts,1e-12);
    elseif k == d12
        yy = ((3/64)*A_tot)  / max(Ts,1e-12);
    elseif k == d13
        yy = ((1/64)*A_tot)  / max(Ts,1e-12);
    elseif k == d14
        yy = ((3/64)*A_tot)  / max(Ts,1e-12);
    elseif k == d15
        yy = ((3/64)*A_tot)  / max(Ts,1e-12);
    elseif k == d16
        yy = ((1/64)*A_tot)  / max(Ts,1e-12);
    end

    k = k + double(1);
    if k > d16 + double(1)
        armed = false;
    end
end

== matlab function iscrt/control signal ==
  data: rpm input; spr input; dir input
function spdcntrldrv(rpm, spr, dir)
a = arduino(); 

dirPin = 'D2'; 
stepPin = 'D3'; 

configurePin(a, dirPin, 'DigitalOutput');
configurePin(a, stepPin, 'DigitalOutput');

stepDelay = 60 / (spr * rpm); 

if dir == 1
    writeDigitalPin(a, dirPin, 1);  % CW
    for i = 1:stepsPerRev
        writeDigitalPin(a, stepPin, 1);
        pause(stepDelay/2);
        writeDigitalPin(a, stepPin, 0);
        pause(stepDelay/2);
    end
else
    writeDigitalPin(a, dirPin, 0);  % CCW
    for i = 1:stepsPerRev
        writeDigitalPin(a, stepPin, 1);
        pause(stepDelay/2);
        writeDigitalPin(a, stepPin, 0);
        pause(stepDelay/2);
    end
end

== matlab function iscrt/ZVZV Shaper/Shaper ==
  data: u input; yy output; Ts input; wn1 input; wn2 input
function yy = ZVZVshaper(u, Ts, wn1, wn2)

persistent armed k last_u A_tot d2 d3 d4
if isempty(armed)
    armed  = false;
    k      = double(0);
    last_u = 0.0;
    A_tot  = 0.0;
    d2     = double(0);
    d3     = double(0);
    d4     = double(0);
end

yy = 0.0;                
tol = 1e-12;

du = u - last_u;
last_u = u;

if ~armed && (abs(du) > tol)
    A_tot = du;
    k     = double(0);
    T1    = 2*pi / max(wn1, 1e-9);
    T2    = 2*pi / max(wn2, 1e-9);
    d2    = double( round( (0.5*T2) / max(Ts,1e-12) ) ); 
    d3    = double( round( (0.5*T1) / max(Ts,1e-12) ) );
    d4    = double( round( (0.5*(T1 + T2)) / max(Ts,1e-12) ) );
    armed = true;
end


if armed
    if k == double(0)
        yy = (0.25*A_tot)  / max(Ts,1e-12);
    elseif k == d2
        yy = (0.25*A_tot)  / max(Ts,1e-12);
    elseif k == d3
        yy = (0.25*A_tot)  / max(Ts,1e-12);
    elseif k == d4
        yy = (0.25*A_tot)  / max(Ts,1e-12);
    end

    k = k + double(1);
    if k > d4 + double(1)
        armed = false;
    end
end

== matlab function iscrt/ZVZVD Shaper/Periodize ==
  data: lh input; ll input; mh input; wn1 output; wn2 output; ml input
function [wn1, wn2]= ModePeriodize(lh, ll, mh, ml)

g = 9.81;

a = mh * lh * ll;
b = (mh * g * ll) + (ml * g * ll) + (mh * g * lh) + (ml * g * lh);
c = (mh * g * g) + (ml * g * g);

wn1 = sqrt((b - sqrt(b * b - 4 * a * c))/ (2 * a));
wn2 = sqrt((b + sqrt(b * b - 4 * a * c))/ (2 * a));

== matlab function iscrt/ZVZVD Shaper/Shaper ==
  data: u input; yy output; Ts input; wn1 input; wn2 input
function yy = ZVZVshaper(u, Ts, wn1, wn2)

persistent armed k last_u A_tot d2 d3 d4 d5 d6
if isempty(armed)
    armed  = false;
    k      = double(0);
    last_u = 0.0;
    A_tot  = 0.0;
    d2     = double(0);
    d3     = double(0);
    d4     = double(0);
    d5     = double(0);
    d6     = double(0);
end

yy = 0.0;                
tol = 1e-12;

du = u - last_u;
last_u = u;

if ~armed && (abs(du) > tol)
    A_tot = du;
    k     = double(0);
    T1    = 2*pi / max(wn1, 1e-9);
    T2    = 2*pi / max(wn2, 1e-9);
    d2    = double( round( (0.5*T2) / max(Ts,1e-12) ) ); 
    d3    = double( round( T2 / max(Ts,1e-12) ) );
    d4    = double( round( (0.5*T1) / max(Ts,1e-12) ) );
    d5    = double( round( (0.5*(T1+T2)) / max(Ts,1e-12) ) );
    d6    = double( round( (0.5*T1+T2) / max(Ts,1e-12) ) );
    armed = true;
end


if armed
    if k == double(0)
        yy = (0.125*A_tot)  / max(Ts,1e-12);
    elseif k == d2
        yy = (0.25*A_tot)  / max(Ts,1e-12);
    elseif k == d3
        yy = (0.125*A_tot)  / max(Ts,1e-12);
    elseif k == d4
        yy = (0.125*A_tot)  / max(Ts,1e-12);
    elseif k == d5
        yy = (0.25*A_tot)  / max(Ts,1e-12);
    elseif k == d6
        yy = (0.125*A_tot)  / max(Ts,1e-12);
    end

    k = k + double(1);
    if k > d6 + double(1)
        armed = false;
    end
end

== matlab function iscrt/ZVZVDD Shaper/Periodize ==
  data: lh input; ll input; mh input; wn1 output; wn2 output; ml input
function [wn1, wn2]= ModePeriodize(lh, ll, mh, ml)

g = 9.81;

a = mh * lh * ll;
b = (mh * g * ll) + (ml * g * ll) + (mh * g * lh) + (ml * g * lh);
c = (mh * g * g) + (ml * g * g);

wn1 = sqrt((b - sqrt(b * b - 4 * a * c))/ (2 * a));
wn2 = sqrt((b + sqrt(b * b - 4 * a * c))/ (2 * a));

== matlab function iscrt/ZVZVDD Shaper/Shaper ==
  data: u input; yy output; Ts input; wn1 input; wn2 input
function yy = ZVZVshaper(u, Ts, wn1, wn2)

persistent armed k last_u A_tot d2 d3 d4 d5 d6 d7 d8
if isempty(armed)
    armed  = false;
    k      = double(0);
    last_u = 0.0;
    A_tot  = 0.0;
    d2     = double(0);
    d3     = double(0);
    d4     = double(0);
    d5     = double(0);
    d6     = double(0);
    d7     = double(0);
    d8     = double(0);
end

yy = 0.0;                
tol = 1e-12;

du = u - last_u;
last_u = u;

if ~armed && (abs(du) > tol)
    A_tot = du;
    k     = double(0);
    T1    = 2*pi / max(wn1, 1e-9);
    T2    = 2*pi / max(wn2, 1e-9);
    d2    = double( round( (0.5*T2) / max(Ts,1e-12) ) ); 
    d3    = double( round( T2 / max(Ts,1e-12) ) );
    d4    = double( round( (1.5*T2) / max(Ts,1e-12) ) );
    d5    = double( round( (0.5*T2) / max(Ts,1e-12) ) );
    d6    = double( round( (0.5*(T1+T2)) / max(Ts,1e-12) ) );
    d7    = double( round( (0.5*T1+T2) / max(Ts,1e-12) ) );
    d8    = double( round( ((0.5*T1)+(1.5*T2)) / max(Ts,1e-12) ) );
    armed = true;
end


if armed
    if k == double(0)
        yy = ((1/16)*A_tot)  / max(Ts,1e-12);
    elseif k == d2
        yy = ((3/16)*A_tot)  / max(Ts,1e-12);
    elseif k == d3
        yy = ((3/16)*A_tot)  / max(Ts,1e-12);
    elseif k == d4
        yy = ((1/16)*A_tot)  / max(Ts,1e-12);
    elseif k == d5
        yy = ((1/16)*A_tot)  / max(Ts,1e-12);
    elseif k == d6
        yy = ((3/16)*A_tot)  / max(Ts,1e-12);
    elseif k == d7
        yy = ((3/16)*A_tot)  / max(Ts,1e-12);
    elseif k == d8
        yy = ((1/16)*A_tot)  / max(Ts,1e-12);
    end

    k = k + double(1);
    if k > d8 + double(1)
        armed = false;
    end
end

== matlab function iscrt/ZVDZV Shaper/Periodize ==
  data: lh input; ll input; mh input; wn1 output; wn2 output; ml input
function [wn1, wn2]= ModePeriodize(lh, ll, mh, ml)

g = 9.81;

a = mh * lh * ll;
b = (mh * g * ll) + (ml * g * ll) + (mh * g * lh) + (ml * g * lh);
c = (mh * g * g) + (ml * g * g);

wn1 = sqrt((b - sqrt(b * b - 4 * a * c))/ (2 * a));
wn2 = sqrt((b + sqrt(b * b - 4 * a * c))/ (2 * a));

== matlab function iscrt/ZVDZV Shaper/Shaper ==
  data: u input; yy output; Ts input; wn1 input; wn2 input
function yy = ZVZVshaper(u, Ts, wn1, wn2)

persistent armed k last_u A_tot d2 d3 d4 d5 d6 d7 d8
if isempty(armed)
    armed  = false;
    k      = double(0);
    last_u = 0.0;
    A_tot  = 0.0;
    d2     = double(0);
    d3     = double(0);
    d4     = double(0);
    d5     = double(0);
    d6     = double(0);
    d7     = double(0);
    d8     = double(0);
end

yy = 0.0;                
tol = 1e-12;

du = u - last_u;
last_u = u;

if ~armed && (abs(du) > tol)
    A_tot = du;
    k     = double(0);
    T1    = 2*pi / max(wn1, 1e-9);
    T2    = 2*pi / max(wn2, 1e-9);
    d2    = double( round( (0.5*T2) / max(Ts,1e-12) ) ); 
    d3    = double( round( (0.5*T1) / max(Ts,1e-12) ) );
    d4    = double( round( (0.5*(T1+T2)) / max(Ts,1e-12) ) );
    d5    = double( round( T1 / max(Ts,1e-12) ) );
    d6    = double( round( (0.5*T2+T1) / max(Ts,1e-12) ) );
    armed = true;
end


if armed
    if k == double(0)
        yy = ((1/8)*A_tot)  / max(Ts,1e-12);
    elseif k == d2
        yy = ((1/8)*A_tot)  / max(Ts,1e-12);
    elseif k == d3
        yy = ((2/8)*A_tot)  / max(Ts,1e-12);
    elseif k == d4
        yy = ((2/8)*A_tot)  / max(Ts,1e-12);
    elseif k == d5
        yy = ((1/8)*A_tot)  / max(Ts,1e-12);
    elseif k == d6
        yy = ((1/8)*A_tot)  / max(Ts,1e-12);
    end

    k = k + double(1);
    if k > d6 + double(1)
        armed = false;
    end
end

== matlab function iscrt/ZVDZVD Shaper/Periodize ==
  data: lh input; ll input; mh input; wn1 output; wn2 output; ml input
function [wn1, wn2]= ModePeriodize(lh, ll, mh, ml)

g = 9.81;

a = mh * lh * ll;
b = (mh * g * ll) + (ml * g * ll) + (mh * g * lh) + (ml * g * lh);
c = (mh * g * g) + (ml * g * g);

wn1 = sqrt((b - sqrt(b * b - 4 * a * c))/ (2 * a));
wn2 = sqrt((b + sqrt(b * b - 4 * a * c))/ (2 * a));
